simulink model "model7_1"  (R2024b)
settings: Solver=VariableStepAuto  StartTime=0.0  StopTime=10.0  RelTol=1e-3
libraries: simulink x1
settings Model: Creator=ryandavis  LastModifiedBy=ryandavis

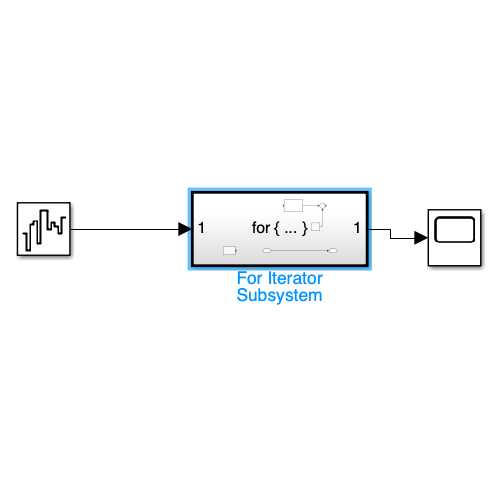
[thumbnail: Simulink's stored preview of the top-level diagram]
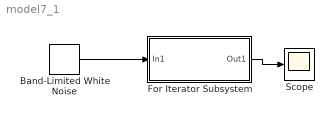
== system model7_1 ==
  Band-Limited White Noise : simulink/Sources/Band-Limited White Noise  Cov=[0.1]  Ts=0.1  seed=[23341]
  For Iterator Subsystem : Subsystem  TreatAsAtomicUnit=on
  Scope : Scope
  wires:
  For Iterator Subsystem/1(Out1) -> Scope/1
  Band-Limited White Noise/1 -> For Iterator Subsystem/1(In1)

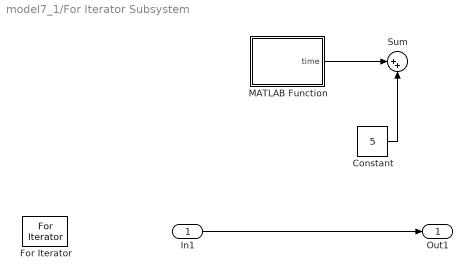
== system model7_1/For Iterator Subsystem ==
  In1 : Inport
  Constant : Constant  Value=5
  For Iterator : ForIterator  IterationLimit=4
  MATLAB Function : MATLAB Function  TreatAsAtomicUnit=on
  Sum : Sum  Inputs=|++
  Out1 : Outport
  wires:
  In1/1 -> Out1/1
  MATLAB Function/1(time) -> Sum/1
  Constant/1 -> Sum/2

== matlab function model7_1/For Iterator Subsystem/MATLAB Function ==
  data: time output
function time = SelectPath()
    persistent minTime maxTime totalTime count;

    if isempty(minTime)
        minTime = Inf;    
        maxTime = -Inf;   
        totalTime = 0;    
        count = 0;        
    end

    r = rand();

    if r < 0.2
        selectedTime = 10;
    elseif r < 0.7
        selectedTime = 20;
    elseif r < 0.8
        selectedTime = 30;
    else
        selectedTime = 40;
    end

    time = selectedTime + 5;

    minTime = min(minTime, min([10, 20, 30, 40]) + 5);
    maxTime = max(maxTime, max([10, 20, 30, 40]) + 5);
    totalTime = totalTime + time;
    count = count + 1;

    avgTime = totalTime / count;

    fprintf('Current Time: %.2f, Min Time: %.2f, Max Time: %.2f, Avg Time: %.2f\n', ...
            time, minTime, maxTime, avgTime);
end
